simulink model "sml_bicycle"  (R2016a)
settings: Solver=VariableStepAuto  StartTime=0.0  StopTime=10.0  RelTol=1e-3
libraries: simulink x2
settings Model: Creator=Duy Nam  LastModifiedBy=Duy Nam

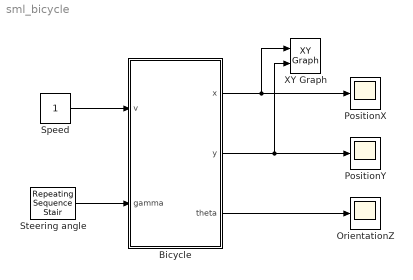
== system sml_bicycle ==
  Bicycle : Subsystem
  OrientationZ : Scope
  PositionX : Scope
  PositionY : Scope
  Speed : Constant
  Steering angle : simulink/Sources/Repeating Sequence Stair  OutValues=[0 0 0 0.5 0 -0.5 0 0 0 0]  tsamp=1  OutMin=[]  OutMax=[]  OutDataTypeStr=double  OutputDataTypeScalingMode=Specify via dialog  OutDataType=double  ConRadixGroup=Best Precision: Vector-wise  OutScaling=2^-12
  XY Graph : simulink/Sinks/XY Graph  xmin=0  xmax=10  ymin=0  ymax=10  st=-1
  wires:
  Speed/1 -> Bicycle/1(v)
  Steering angle/1 -> Bicycle/2(gamma)
  Bicycle/1(x) -> PositionX/1, XY Graph/1
  Bicycle/2(y) -> PositionY/1, XY Graph/2
  Bicycle/3(theta) -> OrientationZ/1

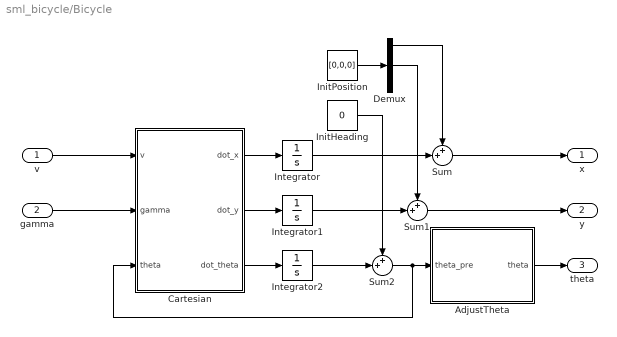
== system sml_bicycle/Bicycle ==
  v : Inport
  gamma : Inport  Port=2
  AdjustTheta : MATLAB Function  TreatAsAtomicUnit=on
  Cartesian : MATLAB Function  TreatAsAtomicUnit=on
  Demux : Demux  Outputs=3
  InitHeading : Constant  Value=0
  InitPosition : Constant  Value=[0,0,0]
  Integrator : Integrator
  Integrator1 : Integrator
  Integrator2 : Integrator
  Sum : Sum  Inputs=++|
  Sum1 : Sum  Inputs=++|
  Sum2 : Sum  Inputs=++|
  x : Outport
  y : Outport  Port=2
  theta : Outport  Port=3
  wires:
  Cartesian/1(dot_x) -> Integrator/1
  Integrator/1 -> Sum/2
  Cartesian/2(dot_y) -> Integrator1/1
  Integrator1/1 -> Sum1/2
  Cartesian/3(dot_theta) -> Integrator2/1
  AdjustTheta/1(theta) -> theta/1
  Sum2/1 -> Cartesian/3(theta), AdjustTheta/1(theta_pre)
  v/1 -> Cartesian/1(v)
  gamma/1 -> Cartesian/2(gamma)
  InitPosition/1 -> Demux/1
  Sum/1 -> x/1
  Demux/1 -> Sum/1
  Sum1/1 -> y/1
  Demux/2 -> Sum1/1
  Integrator2/1 -> Sum2/2
  InitHeading/1 -> Sum2/1

== matlab function sml_bicycle/Bicycle/AdjustTheta ==
  data: theta_pre input; theta output
function theta = AdjustTheta(theta_pre)
% ADJUSTTHETA Adjust the heading angle always between [-pi/2;pi/2]
%% INPUTS
% theta_pre = The heading angle before adjust
%% OUTPUTS
% theta = The heading angle after adjust
%% AdjustTheta
theta = theta_pre - 2*pi*floor((theta_pre + pi)/(2*pi));
end

== matlab function sml_bicycle/Bicycle/Cartesian ==
  data: dot_x output; dot_y output; v input; gamma input; theta input; dot_theta output
function [dot_x, dot_y, dot_theta] = Cartesian(v, gamma, theta)
% CARTESIAN Compute the velocity of robot in world frame
%% INPUTS
% v     = The velocity of the back wheel
% gamma = The steering wheel angle
% theta = The heading angle
%% OUTPUTS
% dot_x     = The velocity of robot in world frame x-axis
% dot_y     = The velocity of robot in world frame y-axis
% dot theta = The rate of change of heading
%% PARAMETERS
L = params_bicycle();
%% Cartesian
dot_x = v*cos(theta);
dot_y = v*sin(theta);
dot_theta = v/L*tan(gamma);
end
